simulink model "Clik_Jacobian_inverse"  (R2023b)
settings: Solver=VariableStepAuto  StartTime=0.0  StopTime=20  RelTol=1e-3
model workspace: external: MAT-File (data not in the file)
undefined symbols (not defined in the file): DiscIntNeverNeededParam, f_s
settings Model: Creator=benit  LastModifiedBy=ANDREA
settings OptimizationCC: ReuseModelBlockBuffer=off

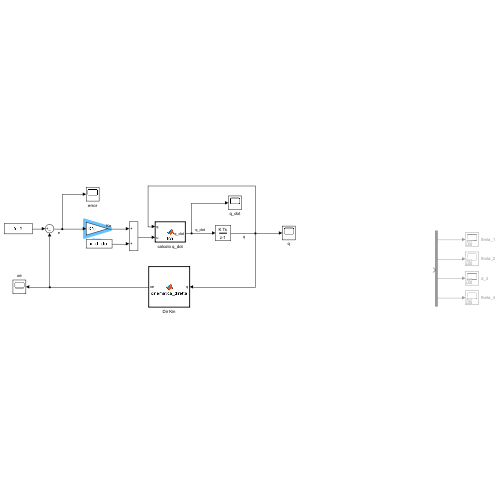
[thumbnail: Simulink's stored preview of the top-level diagram]
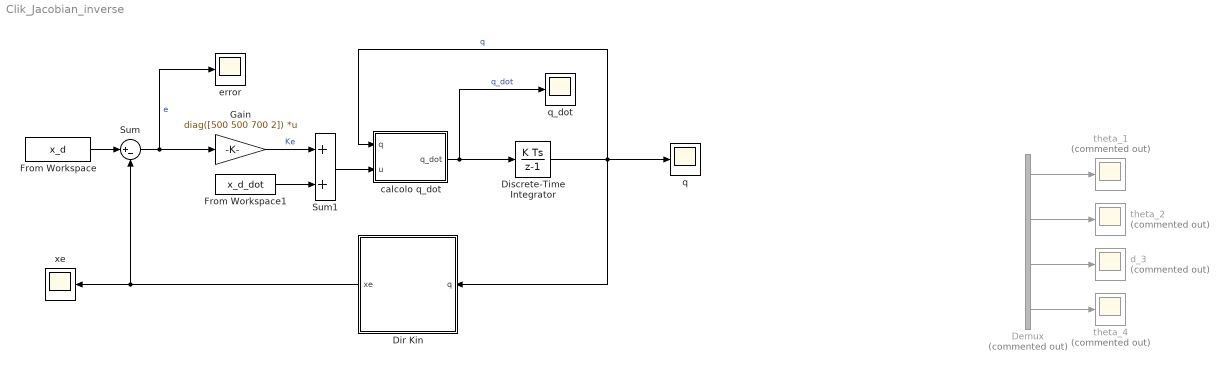
== system Clik_Jacobian_inverse ==
  Demux : Demux  Commented=on
  Dir Kin : MATLAB Function  TreatAsAtomicUnit=on
  Discrete-Time Integrator : DiscreteIntegrator  gainval=1  InitialCondition=config_p_init'  SampleTime=1/f_s  ICPrevOutput=DiscIntNeverNeededParam  ICPrevScaledInput=DiscIntNeverNeededParam
  From Workspace : FromWorkspace  VariableName=x_d
  From Workspace1 : FromWorkspace  VariableName=x_d_dot
  Gain : Gain  Gain=diag([500 500 700 2])  Multiplication=Matrix(K*u)
  Sum : Sum  Inputs=|+-
  Sum1 : Sum
  calcolo q_dot : MATLAB Function  TreatAsAtomicUnit=on
  d_3 : Scope  Commented=on
  error : Scope
  q : Scope
  q_dot : Scope
  theta_1 : Scope  Commented=on
  theta_2 : Scope  Commented=on
  theta_4 : Scope  Commented=on
  xe : Scope
  wires:
  Gain/1 -> Sum1/1  "Ke"
  Sum/1 -> error/1, Gain/1  "e"
  Demux/1 -> theta_1/1
  Demux/2 -> theta_2/1
  Demux/3 -> d_3/1
  From Workspace/1 -> Sum/1
  Discrete-Time Integrator/1 -> q/1, Dir Kin/1(q), calcolo q_dot/1(q)  "q"
  calcolo q_dot/1(q_dot) -> q_dot/1, Discrete-Time Integrator/1  "q_dot"
  Sum1/1 -> calcolo q_dot/2(u)
  Dir Kin/1(xe) -> xe/1, Sum/2
  From Workspace1/1 -> Sum1/2
  Demux/4 -> theta_4/1

== matlab function Clik_Jacobian_inverse/calcolo q_dot ==
  data: q input; u input; q_dot output
function q_dot = fcn(q,u)

    J = [-0.5*sin(q(1))-0.5*sin(q(1)+q(2))   -0.5*sin(q(1)+q(2))    0  0 
          0.5*cos(q(1))+0.5*cos(q(1)+q(2))    0.5*cos(q(1)+q(2))    0  0 
          0                                   0                    -1  0
          1                                   1                     0  -1];
    
    q_dot = pinv(J)*u;

end

== matlab function Clik_Jacobian_inverse/Dir Kin ==
  data: q input; xe output
function xe = cinematica_diretta(q)
    
    xe = [  0.5*cos(q(1))+0.5*cos(q(1)+q(2));
            0.5*sin(q(1))+0.5*sin(q(1)+q(2));
            1/2-q(3)
            q(1)+q(2)-q(4) ];

end
